simulink model "isiprojectsimulink"  (R2022b)
settings: Solver=VariableStepAuto  StartTime=0.0  StopTime=10  RelTol=1e-3
values from neighbouring files (symbols this model uses):
  a = 87.25    [condizione iniziali.mat]    (also in init.m)
  b = 40.77    [condizione iniziali.mat]    (also in init.m)
  c = 67    [condizione iniziali.mat]    (also in init.m)
  d = 0.4    [condizione iniziali.mat]    (also in init.m)
  IAy = 0.025    [condizione iniziali.mat]    (also in init.m)
  IAz = 7    [condizione iniziali.mat]    (also in init.m)
  IGz = 7.5    [condizione iniziali.mat]    (also in init.m)
  IPy = 0.045    [condizione iniziali.mat]    (also in init.m)
  IPz = 3.5    [condizione iniziali.mat]    (also in init.m)
  L = Pxy*S^(-1)    [UKF_filter.m]    (also in UKF_filter_Diff_Periodi.m; condizione iniziali.mat = 1.5; init.m = 1.5)
  l = 0.8    [condizione iniziali.mat]    (also in init.m)
  ma = 2    [condizione iniziali.mat]    (also in init.m)
  mp = 2    [condizione iniziali.mat]    (also in init.m)
  Mv = 80    [condizione iniziali.mat]    (also in init.m)
  phi_dot_0 = 0    [condizione iniziali.mat]    (also in init.m)
  psi_dot_0 = 0    [condizione iniziali.mat]    (also in init.m)
  ra = 0.2    [condizione iniziali.mat]    (also in init.m)
  rp = 0.2    [condizione iniziali.mat]    (also in init.m)
  sensor_var = 0    [condizione iniziali.mat]    (also in init.m)
  t_sample = 0.1    [condizione iniziali.mat]    (also in init.m)
  theta_0 = 2.65000429413    [condizione iniziali.mat]    (also in init.m = 2*pi*rand(1))
  x_0 = 8.00280468889    [condizione iniziali.mat]    (also in init.m = limits * rand(1))
  y_0 = 1.41886338627    [condizione iniziali.mat]    (also in init.m = limits * rand(1))
undefined symbols (not defined in the file or in its folder): sigbuilder_block
libraries: simulink x2
settings Model: Creator=Marco  LastModifiedBy=39327
settings ModelReferenceCC: EnableRefExpFcnMdlSchedulingChecks=on

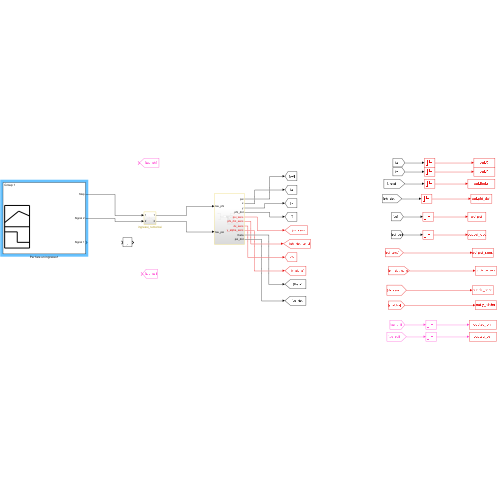
[thumbnail: Simulink's stored preview of the top-level diagram]
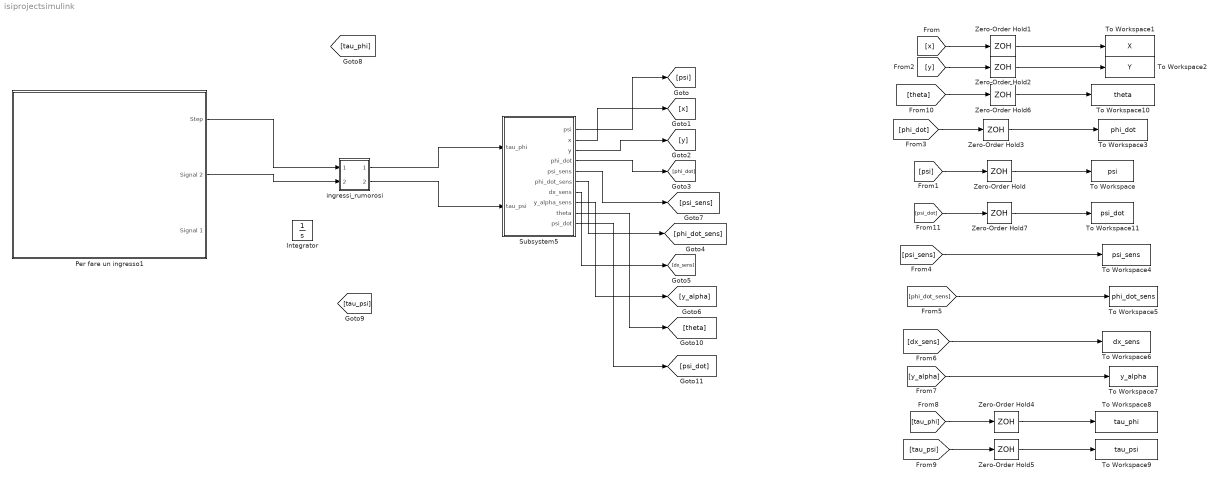
== system isiprojectsimulink ==
  Integrator : Integrator
  Per fare un ingresso1 : Subsystem  Tag=STV Subsys  LoadFcn=sigbuilder_block('load');  StartFcn=sigbuilder_block('start');  StopFcn=sigbuilder_block('stop');  ClipboardFcn=sigbuilder_block('clipboard');  mask(Sigbuilder block){tuvar=[0:10]}
      mask help: Simulink:masks:SigbuilderBlock_MD
      mask init:
      | if ~strcmp(get_param(bdroot(gcbh),'SimulationStatus'),'stopped') tuvar = sigbuilder_block('maskInit'); end
      settings: CopyFcn=sigbuilder_block('copy');  DeleteFcn=sigbuilder_block('delete');  ModelCloseFcn=sigbuilder_block('modelClose');  PreSaveFcn=sigbuilder_block('preSave');  PauseFcn=sigbuilder_block('pause');  ContinueFcn=sigbuilder_block('continue');  NameChangeFcn=sigbuilder_block('namechange');  OpenFcn=sigbuilder_block('open',[5.4 42.6 949.1 432.4 ]);  CloseFcn=sigbuilder_block('close');
      mask Display: plot(0, 0, 100, 100,[2, 2, 32, 32, 2], [68, 8, 8, 68, 68],[32, 2], [38, 38], [32, 19, 2],[53, 60, 44], [32, 17, 17, 2],[16, 16, 31, 31]);txt = getActiveGroup(gcbh);text(2, 100, txt,'verticalAlignment', 'top');
  Subsystem5 : Subsystem
  To Workspace : ToWorkspace  VariableName=psi  SampleTime=t_sample
      settings: Save2DSignal=2-D array (concatenate along first dimension)
  To Workspace1 : ToWorkspace  VariableName=X  SampleTime=t_sample
      settings: Save2DSignal=2-D array (concatenate along first dimension)
  To Workspace10 : ToWorkspace  VariableName=theta  SampleTime=t_sample
      settings: Save2DSignal=2-D array (concatenate along first dimension)
  To Workspace11 : ToWorkspace  VariableName=psi_dot  SampleTime=t_sample
      settings: Save2DSignal=2-D array (concatenate along first dimension)
  To Workspace2 : ToWorkspace  VariableName=Y  SampleTime=t_sample
      settings: Save2DSignal=2-D array (concatenate along first dimension)
  To Workspace3 : ToWorkspace  VariableName=phi_dot  SampleTime=t_sample
      settings: Save2DSignal=2-D array (concatenate along first dimension)
  To Workspace4 : ToWorkspace  VariableName=psi_sens  SampleTime=t_sample
      settings: Save2DSignal=2-D array (concatenate along first dimension)
  To Workspace5 : ToWorkspace  VariableName=phi_dot_sens  SampleTime=t_sample
      settings: Save2DSignal=2-D array (concatenate along first dimension)
  To Workspace6 : ToWorkspace  VariableName=dx_sens  SampleTime=t_sample
      settings: Save2DSignal=2-D array (concatenate along first dimension)
  To Workspace7 : ToWorkspace  VariableName=y_alpha  SampleTime=t_sample
  To Workspace8 : ToWorkspace  VariableName=tau_phi  SampleTime=t_sample
      settings: Save2DSignal=2-D array (concatenate along first dimension)
  To Workspace9 : ToWorkspace  VariableName=tau_psi  SampleTime=t_sample
      settings: Save2DSignal=2-D array (concatenate along first dimension)
  Zero-Order Hold{,1..7} (8 alike) : ZeroOrderHold  SampleTime=-1
  ingressi_rumorosi : Subsystem
  wires:
  Subsystem5/8(y_alpha_sens) -> [y_alpha]
  Subsystem5/5(psi_sens) -> [psi_sens]
  Subsystem5/1(psi) -> [psi]
  Subsystem5/2(x) -> [x]
  Subsystem5/3(y) -> [y]
  Subsystem5/4(phi_dot) -> [phi_dot]
  Subsystem5/6(phi_dot_sens) -> [phi_dot_sens]
  Subsystem5/7(dx_sens) -> [dx_sens]
  ingressi_rumorosi/1(Out1) -> Subsystem5/1(tau_phi)
  ingressi_rumorosi/2(Out2) -> Subsystem5/2(tau_psi)
  [y_alpha] -> To Workspace7/1
  [dx_sens] -> To Workspace6/1
  Zero-Order Hold4/1 -> To Workspace8/1
  [psi] -> Zero-Order Hold/1
  [phi_dot_sens] -> To Workspace5/1
  Zero-Order Hold5/1 -> To Workspace9/1
  [y] -> Zero-Order Hold2/1
  Zero-Order Hold/1 -> To Workspace/1
  [psi_sens] -> To Workspace4/1
  Zero-Order Hold3/1 -> To Workspace3/1
  [tau_phi] -> Zero-Order Hold4/1
  Zero-Order Hold1/1 -> To Workspace1/1
  [phi_dot] -> Zero-Order Hold3/1
  Zero-Order Hold2/1 -> To Workspace2/1
  [x] -> Zero-Order Hold1/1
  [tau_psi] -> Zero-Order Hold5/1
  Subsystem5/9(theta) -> [theta]
  [theta] -> Zero-Order Hold6/1
  Zero-Order Hold6/1 -> To Workspace10/1
  Subsystem5/10(psi_dot) -> [psi_dot]
  [psi_dot] -> Zero-Order Hold7/1
  Zero-Order Hold7/1 -> To Workspace11/1
  Per fare un ingresso1/1(Step) -> ingressi_rumorosi/1(In1)
  Per fare un ingresso1/2(Signal 2) -> ingressi_rumorosi/2(In2)

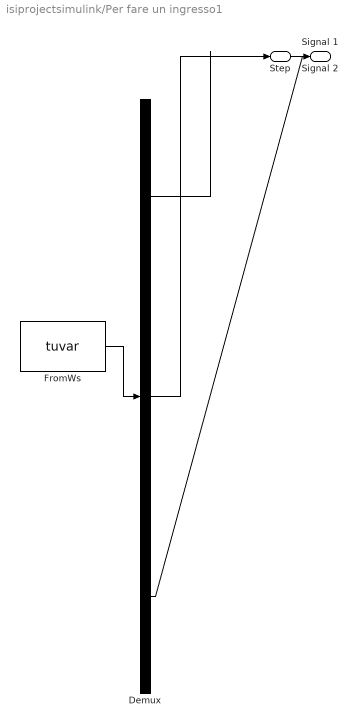
== system isiprojectsimulink/Per fare un ingresso1 ==
  Demux : Demux  Tag=STV Demux  Outputs=3
      settings: DisplayOption=none
  FromWs : FromWorkspace  Tag=STV FromWs  VariableName=tuvar
      SigBuilderData=|
      | common.afterFinalStr = 'Extrapolate'
      | common.sampleTime = 0
      | dataSet.timeRange = [0 10]
      | dataSet.name = 'Group 1'
      | sbobj.Groups.Name = 'Group 1'
      | sbobj.Groups.Signals(1).Name = 'Step'
      | sbobj.Groups.Signals(1).XData = [0 5 5 10]
      | sbobj.Groups.Signals(1).YData = [0 0 0.005 0.005]
      | sbobj.Groups.Signals(2).Name = 'Signal 2'
      | sbobj.Groups.Signals(2).XData = [0 4 4 4.001 4.001 10]
      | sbobj.Groups.Signals(2).YData = [0 0 0.0052 0.0052 0 0]
      | sbobj.Groups.Signals(3).Name = 'Signal 1'
      | sbobj.Groups.Signals(3).XData = [0 5 5 10]
      | sbobj.Groups.Signals(3).YData = [0 0 0.3 0.3]
  Step : Outport  Tag=STV Outport
  Signal 2 : Outport  Tag=STV Outport  Port=2
  Signal 1 : Outport  Tag=STV Outport  Port=3
  wires:
  FromWs/1 -> Demux/1
  Demux/1 -> Step/1
  Demux/2 -> Signal 2/1
  Demux/3 -> Signal 1/1

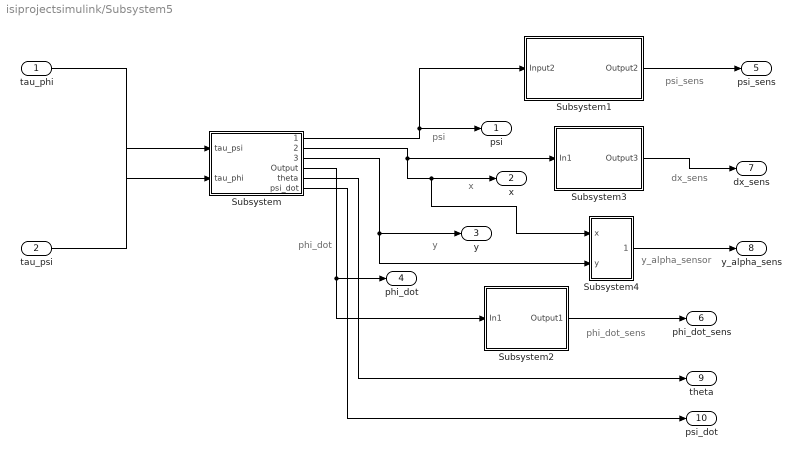
== system isiprojectsimulink/Subsystem5 ==
  note: y_alpha_sensor
  note: phi_dot
  note: y
  note: x
  note: psi
  note: dx_sens
  note: phi_dot_sens
  note: psi_sens
  tau_phi : Inport
  tau_psi : Inport  Port=2
  Subsystem : Subsystem
  Subsystem1 : Subsystem
  Subsystem2 : Subsystem
  Subsystem3 : Subsystem
  Subsystem4 : Subsystem
  psi : Outport
  x : Outport  Port=2
  y : Outport  Port=3
  phi_dot : Outport  Port=4
  psi_sens : Outport  Port=5
  phi_dot_sens : Outport  Port=6
  dx_sens : Outport  Port=7
  y_alpha_sens : Outport  Port=8
  theta : Outport  Port=9
  psi_dot : Outport  Port=10
  wires:
  Subsystem/1(1) -> psi/1, Subsystem1/1(Input2)
  Subsystem/3(3) -> y/1, Subsystem4/2(y)
  Subsystem2/1(Output1) -> phi_dot_sens/1
  Subsystem/4(Output) -> phi_dot/1, Subsystem2/1(In1)
  Subsystem/2(2) -> x/1, Subsystem4/1(x), Subsystem3/1(In1)
  Subsystem1/1(Output2) -> psi_sens/1
  Subsystem3/1(Output3) -> dx_sens/1
  Subsystem4/1(Out1) -> y_alpha_sens/1
  tau_phi/1 -> Subsystem/2(tau_phi)
  tau_psi/1 -> Subsystem/1(tau_psi)
  Subsystem/5(theta) -> theta/1
  Subsystem/6(psi_dot) -> psi_dot/1

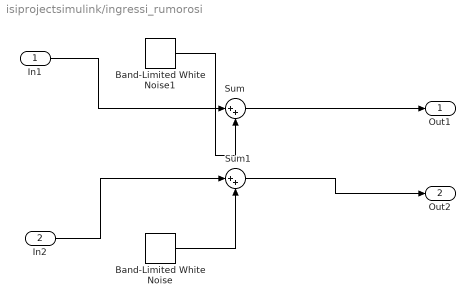
== system isiprojectsimulink/ingressi_rumorosi ==
  In1 : Inport
  In2 : Inport  Port=2
  Band-Limited White Noise : simulink/Sources/Band-Limited White Noise  Cov=[0.1]  Ts=0.1  seed=[23341]
  Band-Limited White Noise1 : simulink/Sources/Band-Limited White Noise  Cov=[0.1]  Ts=0.1  seed=[23341]
  Sum : Sum  Inputs=|++
  Sum1 : Sum  Inputs=|++
  Out1 : Outport
  Out2 : Outport  Port=2
  wires:
  Band-Limited White Noise1/1 -> Sum/2
  In1/1 -> Sum/1
  Band-Limited White Noise/1 -> Sum1/2
  Sum1/1 -> Out2/1
  Sum/1 -> Out1/1
  In2/1 -> Sum1/1

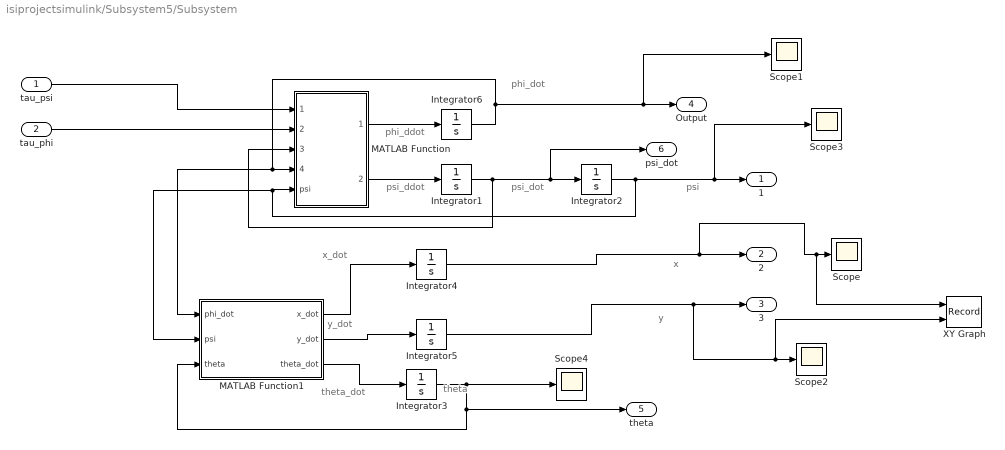
== system isiprojectsimulink/Subsystem5/Subsystem ==
  note: psi
  note: theta_dot
  note: psi_ddot
  note: y_dot
  note: theta
  note: x
  note: x_dot
  note: y
  note: psi_dot
  note: phi_dot
  note: phi_ddot
  tau_psi : Inport
  tau_phi : Inport  Port=2
  Integrator1 : Integrator  InitialCondition=psi_dot_0  IgnoreLimit=on
  Integrator2 : Integrator
  Integrator3 : Integrator  InitialCondition=theta_0  IgnoreLimit=on
  Integrator4 : Integrator  InitialCondition=x_0  IgnoreLimit=on
  Integrator5 : Integrator  InitialCondition=y_0  IgnoreLimit=on
  Integrator6 : Integrator  InitialCondition=phi_dot_0  IgnoreLimit=on
  MATLAB Function : MATLAB Function  TreatAsAtomicUnit=on
  MATLAB Function1 : MATLAB Function  TreatAsAtomicUnit=on
  Scope{,1..4} (5 alike) : Scope
  XY Graph : Record  FileSettingsInternal="{\"entries\":[{\"content\":{\"excelSettings\":{\"content\":{},\"type\":\"Streamout.ExcelSettings\"}},\"type\":\"Streamout.FileSettingStorage\",\"uuid\":\"fdb8a2fc-074c-43c6-a046-bc13c53f2439\"}],\"packageUris\":[\"http://schema.mathworks.com/mf0/streamout_blocks/R2020a\"],\"version\":\"1.0\"}"  Layout=[1 1]  SignalsInternal="{\"entries\":[{\"content\":{\"signals\":[{\"content\":{\"blockPath\":[\"isiprojectsimulink/Subsystem5/Subsystem/XY Graph\"],\"channel\":[],\"dimensions\":[1],\"domain\":\"isiprojectsimulink/Subsystem5/Subsystem/XY Graph\",\"lineColor\":\"#a2142f\",\"plots\":[1],\"port\":1,\"sid\":[\"\"],\"signalID\":6764,\"signalName\":\"Integrator4\"},\"type\":\"RecordBlkView.Signal\",\"uuid\":\"5f03eae9-22d6-4936-a0fa-b841567e22ec\"},{\"content\":{\"blockPath\":[\"isiprojectsimulink/Subsystem5/Subsystem/XY Graph\"],\"channel\":[],\"dimensions\":[1],\"domain\":\"isiprojectsimulink/Subsystem5/Subsystem/XY Graph\",\"lineColor\":\"#139fff\",\"plots\":[1],\"port\":2,\"sid\":[\"\"],\"signalID\":6768,\"signalName\":\"Integrator5\"},\"type\":\"RecordBlkView.Signal\",\"uuid\":\"29cc31ae-e961-4c58-8146-30a02bafb080\"}]},\"type\":\"RecordBlkView.InputSignals\",\"uuid\":\"5008649a-4029-4654-a594-c800f383ac65\"}],\"packageUris\":[\"http://schema.mathworks.com/mf0/streamout_blocks/R2020a\"],\"version\":\"1.0\"}"  VisualizationBindings="{\"xyplotplugin\":{\"info\":[{\"series\":[{\"bindingParametersList\":[{\"parameter\":\"X-Axis\",\"signalID\":6764,\"signalName\":\"Integrator4\"},{\"parameter\":\"Y-Axis\",\"signalID\":6768,\"signalName\":\"Integrator5\"}],\"seriesID\":31912}],\"subplotID\":1}]}}"  CompatibilityTag=XY
  1 : Outport
  2 : Outport  Port=2
  3 : Outport  Port=3
  Output : Outport  Port=4
  theta : Outport  Port=5
  psi_dot : Outport  Port=6
  wires:
  Integrator4/1 -> XY Graph/1, Scope/1, 2/1
  Integrator2/1 -> Scope3/1, 1/1, MATLAB Function1/2(psi), MATLAB Function/5(psi)
  MATLAB Function1/3(theta_dot) -> Integrator3/1
  MATLAB Function1/1(x_dot) -> Integrator4/1
  tau_phi/1 -> MATLAB Function/2(tau_phi)
  Integrator5/1 -> XY Graph/2, Scope2/1, 3/1
  tau_psi/1 -> MATLAB Function/1(tau_psi)
  MATLAB Function1/2(y_dot) -> Integrator5/1
  Integrator3/1 -> MATLAB Function1/3(theta), theta/1, Scope4/1
  MATLAB Function/2(psi_ddot) -> Integrator1/1
  MATLAB Function/1(phi_ddot) -> Integrator6/1
  Integrator6/1 -> MATLAB Function1/1(phi_dot), MATLAB Function/4(phi_dot), Scope1/1, Output/1
  Integrator1/1 -> MATLAB Function/3(psi_dot), psi_dot/1, Integrator2/1

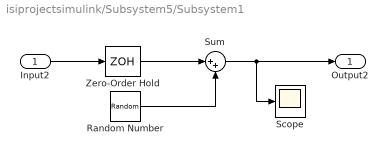
== system isiprojectsimulink/Subsystem5/Subsystem1 ==
  Input2 : Inport
  Random Number : RandomNumber  Variance=sensor_var  SampleTime=t_sample
  Scope : Scope
  Sum : Sum  Inputs=|++
  Zero-Order Hold : ZeroOrderHold  SampleTime=t_sample
  Output2 : Outport
  wires:
  Sum/1 -> Scope/1, Output2/1
  Input2/1 -> Zero-Order Hold/1
  Zero-Order Hold/1 -> Sum/1
  Random Number/1 -> Sum/2

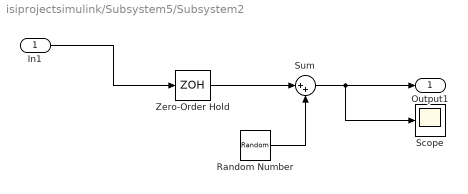
== system isiprojectsimulink/Subsystem5/Subsystem2 ==
  In1 : Inport
  Random Number : RandomNumber  Variance=sensor_var  SampleTime=t_sample
  Scope : Scope
  Sum : Sum  Inputs=|++
  Zero-Order Hold : ZeroOrderHold  SampleTime=t_sample
  Output1 : Outport
  wires:
  Random Number/1 -> Sum/2
  Sum/1 -> Scope/1, Output1/1
  In1/1 -> Zero-Order Hold/1
  Zero-Order Hold/1 -> Sum/1

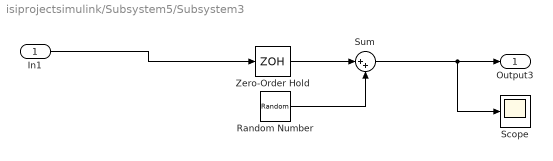
== system isiprojectsimulink/Subsystem5/Subsystem3 ==
  In1 : Inport
  Random Number : RandomNumber  Variance=sensor_var  SampleTime=t_sample
  Scope : Scope
  Sum : Sum  Inputs=|++
  Zero-Order Hold : ZeroOrderHold  SampleTime=t_sample
  Output3 : Outport
  wires:
  Random Number/1 -> Sum/2
  Zero-Order Hold/1 -> Sum/1
  Sum/1 -> Scope/1, Output3/1
  In1/1 -> Zero-Order Hold/1

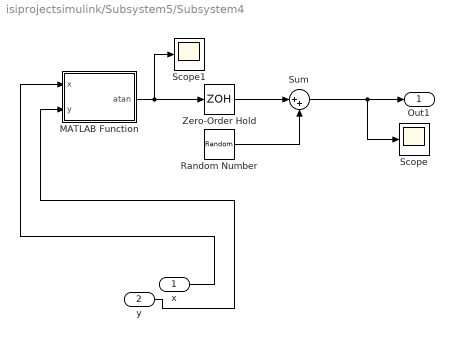
== system isiprojectsimulink/Subsystem5/Subsystem4 ==
  x : Inport
  y : Inport  Port=2
  MATLAB Function : MATLAB Function  TreatAsAtomicUnit=on
  Random Number : RandomNumber  Variance=sensor_var  SampleTime=t_sample
  Scope : Scope
  Scope1 : Scope
  Sum : Sum  Inputs=|++
  Zero-Order Hold : ZeroOrderHold  SampleTime=t_sample
  Out1 : Outport
  wires:
  Sum/1 -> Scope/1, Out1/1
  Random Number/1 -> Sum/2
  Zero-Order Hold/1 -> Sum/1
  MATLAB Function/1(atan) -> Scope1/1, Zero-Order Hold/1
  y/1 -> MATLAB Function/2(y)
  x/1 -> MATLAB Function/1(x)

== matlab function isiprojectsimulink/Subsystem5/Subsystem/MATLAB Function1 ==
  data: phi_dot input; psi input; x_dot output; theta input; y_dot output; rp parameter; L parameter; theta_dot output
function [x_dot,y_dot,theta_dot] = modellocinematico(phi_dot,psi,theta,rp, L)

x_dot = rp*phi_dot*cos(theta)*cos(psi);
y_dot = rp*phi_dot*sin(theta)*cos(psi);
theta_dot = -(rp*phi_dot*sin(psi))/L;

== matlab function isiprojectsimulink/Subsystem5/Subsystem/MATLAB Function ==
  data: phi_ddot output; psi_ddot output; tau_psi input; tau_phi input; psi_dot input; phi_dot input; psi input; a parameter; b parameter; c parameter; rp parameter; l parameter; L parameter; IPy parameter; IPz parameter; Mv parameter; mp parameter; ma parameter; IAy parameter; ra parameter; d parameter; IGz parameter; IAz parameter
function [phi_ddot,psi_ddot]= fcn(tau_psi,tau_phi,psi_dot,phi_dot,psi,a, b, c, rp, l, L, IPy, IPz, Mv, mp, ma, IAy, ra, d, IGz, IAz)
x = psi;

B = [a*rp^2*cos(x)^2+b*(rp/L)^2*sin(x)^2+IPy, -IPz*(rp/L)*sin(x); -IPz*(rp/L)*sin(x), IPz];
C = [(b*(rp/L)^2 - a*rp^2)*phi_dot*psi_dot*sin(x)*cos(x); -IPz*(rp/L)*phi_dot*psi_dot*cos(x)];
%C = [(b*(rp/L)^2 - a*rp^2)*psi_dot*sin(x)*cos(x), (b*(rp/L)^2-a*rp^2)*phi_dot*sin(x)*cos(x)+IPz*(rp/L)*cos(x)*psi_dot; (b*(rp/L)^2-a*rp^2)*phi_dot*sin(x)*cos(x),0];
tau = [ tau_phi;tau_psi];

q=[phi_dot;psi_dot];

M = (inv(B)*(tau-C))';
phi_ddot= M(1);
psi_ddot= M(2);

== matlab function isiprojectsimulink/Subsystem5/Subsystem4/MATLAB Function ==
  data: x input; atan output; y input
function atan   = sensorchoose(x,y)
x = atan2(y,x);
atan = x;
